simulink model "ddc_bpm_476_066"  (Simulink 7.8)
settings: Solver=ode45  StartTime=0.0  StopTime=2e-3  RelTol=1e-3
undefined symbols (not defined in the file): decim_factor_poly_35, dt_sim, frev_476, Fs_adc, n_ch, n_ovs, R_fofb, R_sec, R_sec_cfir, R_sec_pfir, R_tbt, xlipgetpartsetting
libraries: xbsIndex_r4 x1408, simulink x7
(part 8 of 11)

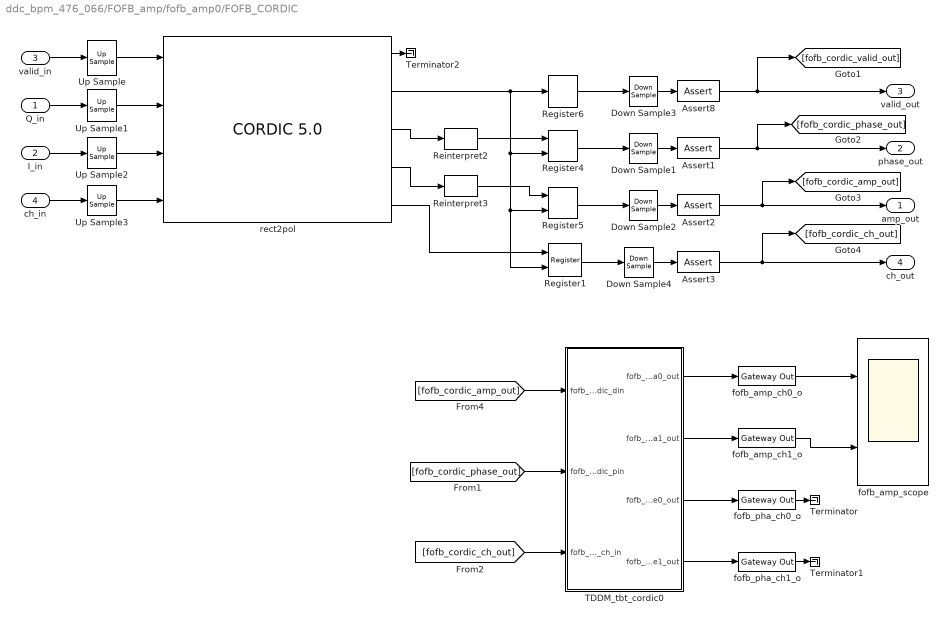
== system ddc_bpm_476_066/FOFB_amp/fofb_amp0/FOFB_CORDIC ==
  Q_in : Inport
  I_in : Inport  Port=2
  valid_in : Inport  Port=3
  ch_in : Inport  Port=4
  Assert{1..3,8} (4 alike) : xbsIndex_r4/Assert  assert_type=off  type_source=Explicitly  gui_display_data_type=Fixed-point  arith_type="Signed  (2's comp)"  n_bits=16  bin_pt=14  preci_type=Single  exp_width=8  frac_width=24  assert_rate=on  rate_source=Explicitly  period=(1/Fs_adc/n_ovs)*R_fofb  output_port=on  block_type=assert
  Down Sample{1..4} (4 alike) : xbsIndex_r4/Down Sample  sample_ratio=R_fofb  sample_phase="Last Value of Frame  (most efficient)"  en=off  latency=1  dbl_ovrd=off  block_type=dsamp
  Register1 : xbsIndex_r4/Register  init=0  rst=off  en=on  dbl_ovrd=off  block_type=register
  Register4 : xbsIndex_r4/Register  init=0  rst=off  en=on  dbl_ovrd=off  block_type=register
  Register5 : xbsIndex_r4/Register  init=0  rst=off  en=on  dbl_ovrd=off  block_type=register
  Register6 : xbsIndex_r4/Register  init=0  rst=off  en=off  dbl_ovrd=off  block_type=register
  Reinterpret2 : xbsIndex_r4/Reinterpret  force_arith_type=off  arith_type=Unsigned  force_bin_pt=off  bin_pt=18  block_type=reinterpret
  Reinterpret3 : xbsIndex_r4/Reinterpret  force_arith_type=off  arith_type=Unsigned  force_bin_pt=off  bin_pt=19  block_type=reinterpret
  TDDM_tbt_cordic0 : Subsystem
  Terminator : Terminator
  Terminator1 : Terminator
  Terminator2 : Terminator
  Up Sample : xbsIndex_r4/Up Sample  sample_ratio=R_fofb  copy_samples=off  en=off  latency=0  dbl_ovrd=off  block_type=usamp
  Up Sample1 : xbsIndex_r4/Up Sample  sample_ratio=R_fofb  copy_samples=on  en=off  latency=0  dbl_ovrd=off  block_type=usamp
  Up Sample2 : xbsIndex_r4/Up Sample  sample_ratio=R_fofb  copy_samples=on  en=off  latency=0  dbl_ovrd=off  block_type=usamp
  Up Sample3 : xbsIndex_r4/Up Sample  sample_ratio=R_fofb  copy_samples=on  en=off  latency=0  dbl_ovrd=off  block_type=usamp
  fofb_amp_ch0_o : xbsIndex_r4/Gateway Out  inherit_from_input=on  hdl_port=on  timing_constraint=Data Rate  locs_specified=off  LOCs={}  UseAsDAC=off  DACChannel='1'  block_type=gatewayout
      settings: infoedit="Gateway out block.  Converts Xilinx fixed-point or floating-point type inputs into ouputs of type Simulink integer, single, double, or fixed point.<br><br>Hardware notes:  In hardware these blocks become top level output ports or are discarded, depending on how they are configured."
  fofb_amp_ch1_o : xbsIndex_r4/Gateway Out  inherit_from_input=on  hdl_port=on  timing_constraint=Data Rate  locs_specified=off  LOCs={}  UseAsDAC=off  DACChannel='1'  block_type=gatewayout
      settings: infoedit="Gateway out block.  Converts Xilinx fixed-point or floating-point type inputs into ouputs of type Simulink integer, single, double, or fixed point.<br><br>Hardware notes:  In hardware these blocks become top level output ports or are discarded, depending on how they are configured."
  fofb_amp_scope : Scope  NumInputPorts=2
      settings: TimeRange=0.00011214  YMin=-0.1~-1.5  YMax=1~1.5  SaveName=ScopeData19  MaxDataPoints=1000000  SampleInput=on
  fofb_pha_ch0_o : xbsIndex_r4/Gateway Out  inherit_from_input=on  hdl_port=on  timing_constraint=Data Rate  locs_specified=off  LOCs={}  UseAsDAC=off  DACChannel='1'  block_type=gatewayout
      settings: infoedit="Gateway out block.  Converts Xilinx fixed-point or floating-point type inputs into ouputs of type Simulink integer, single, double, or fixed point.<br><br>Hardware notes:  In hardware these blocks become top level output ports or are discarded, depending on how they are configured."
  fofb_pha_ch1_o : xbsIndex_r4/Gateway Out  inherit_from_input=on  hdl_port=on  timing_constraint=Data Rate  locs_specified=off  LOCs={}  UseAsDAC=off  DACChannel='1'  block_type=gatewayout
      settings: infoedit="Gateway out block.  Converts Xilinx fixed-point or floating-point type inputs into ouputs of type Simulink integer, single, double, or fixed point.<br><br>Hardware notes:  In hardware these blocks become top level output ports or are discarded, depending on how they are configured."
  rect2pol : xbsIndex_r4/CORDIC 5.0   functional_selection=Translate  architectural_configuration=Word_Serial  pipelining_mode=Optimal  data_format=SignedFraction  phase_format=Radians  input_width=25  output_width=24  round_mode=Nearest_Even  iterations=0  precision=0  compensation_scaling=Embedded_Multiplier  coarse_rotation=on  aclken=off  aresetn=off  out_tready=off  cartesian_has_tuser=on  cartesian_has_tlast=off  cartesian_tuser_width=1  phase_has_tuser=off  phase_has_tlast=off  phase_tuser_width=1  out_tlast_behv=Null  flow_control=NonBlocking  optimize_goal=Resources  trim_axipin_name=on  ip_name=CORDIC  ip_version=5.0  dsptool_ready=true  ipcore_usecache=true  ipcore_useipmodelcache=true  wrapper_available=true  port_translation_map={ 'aclken' => 'en', 'aresetn' => 'rst' }  block_type=cordic_v5_0
      settings: infoedit=CORDIC 5.0
  amp_out : Outport
  phase_out : Outport  Port=2
  valid_out : Outport  Port=3
  ch_out : Outport  Port=4
  wires:
  Register4/1 -> Down Sample1/1
  Register5/1 -> Down Sample2/1
  Register6/1 -> Down Sample3/1
  [fofb_cordic_amp_out] -> TDDM_tbt_cordic0/1(fofb_cordic_din)
  [fofb_cordic_ch_out] -> TDDM_tbt_cordic0/3(fofb_cordic_ch_in)
  Register1/1 -> Down Sample4/1
  TDDM_tbt_cordic0/1(fofb_cordic_data0_out) -> fofb_amp_ch0_o/1
  TDDM_tbt_cordic0/2(fofb_cordic_data1_out) -> fofb_amp_ch1_o/1
  fofb_amp_ch0_o/1 -> fofb_amp_scope/1
  fofb_amp_ch1_o/1 -> fofb_amp_scope/2
  [fofb_cordic_phase_out] -> TDDM_tbt_cordic0/2(fofb_cordic_pin)
  TDDM_tbt_cordic0/3(fofb_cordic_phase0_out) -> fofb_pha_ch0_o/1
  TDDM_tbt_cordic0/4(fofb_cordic_phase1_out) -> fofb_pha_ch1_o/1
  fofb_pha_ch0_o/1 -> Terminator/1
  fofb_pha_ch1_o/1 -> Terminator1/1
  Reinterpret2/1 -> Register4/1
  Reinterpret3/1 -> Register5/1
  rect2pol/2 -> Register5/2, Register1/2, Register4/2, Register6/1
  rect2pol/3 -> Reinterpret2/1
  rect2pol/4 -> Reinterpret3/1
  rect2pol/5 -> Register1/1
  rect2pol/1 -> Terminator2/1
  valid_in/1 -> Up Sample/1
  Q_in/1 -> Up Sample1/1
  I_in/1 -> Up Sample2/1
  ch_in/1 -> Up Sample3/1
  Up Sample/1 -> rect2pol/1
  Up Sample1/1 -> rect2pol/2
  Up Sample2/1 -> rect2pol/3
  Up Sample3/1 -> rect2pol/4
  Down Sample3/1 -> Assert8/1
  Down Sample1/1 -> Assert1/1
  Down Sample2/1 -> Assert2/1
  Down Sample4/1 -> Assert3/1
  Assert8/1 -> valid_out/1, [fofb_cordic_valid_out]
  Assert1/1 -> phase_out/1, [fofb_cordic_phase_out]
  Assert2/1 -> amp_out/1, [fofb_cordic_amp_out]
  Assert3/1 -> ch_out/1, [fofb_cordic_ch_out]

== system ddc_bpm_476_066/FOFB_amp/fofb_amp0/FOFB_amp ==
  Q_in : Inport
  I_in : Inport  Port=2
  ch_in : Inport  Port=3
  Reg : Subsystem
  Reg1 : Subsystem
  TDDM_fofb_cic0 : Subsystem
  cic_fofb : Subsystem
  cic_fofb0_scope : Scope  NumInputPorts=4
      settings: TimeRange=0.00011214  YMin=-0.1~-1.5~-0.002~-1.5  YMax=1~1.5~0.00075~1.5  SaveName=ScopeData18  MaxDataPoints=1000000  SampleInput=on
  fofb_decim_ch0_i_o : xbsIndex_r4/Gateway Out  inherit_from_input=on  hdl_port=on  timing_constraint=Data Rate  locs_specified=off  LOCs={}  UseAsDAC=off  DACChannel='1'  block_type=gatewayout
      settings: infoedit="Gateway out block.  Converts Xilinx fixed-point or floating-point type inputs into ouputs of type Simulink integer, single, double, or fixed point.<br><br>Hardware notes:  In hardware these blocks become top level output ports or are discarded, depending on how they are configured."
  fofb_decim_ch0_q_o : xbsIndex_r4/Gateway Out  inherit_from_input=on  hdl_port=on  timing_constraint=Data Rate  locs_specified=off  LOCs={}  UseAsDAC=off  DACChannel='1'  block_type=gatewayout
      settings: infoedit="Gateway out block.  Converts Xilinx fixed-point or floating-point type inputs into ouputs of type Simulink integer, single, double, or fixed point.<br><br>Hardware notes:  In hardware these blocks become top level output ports or are discarded, depending on how they are configured."
  fofb_decim_ch1_i_o : xbsIndex_r4/Gateway Out  inherit_from_input=on  hdl_port=on  timing_constraint=Data Rate  locs_specified=off  LOCs={}  UseAsDAC=off  DACChannel='1'  block_type=gatewayout
      settings: infoedit="Gateway out block.  Converts Xilinx fixed-point or floating-point type inputs into ouputs of type Simulink integer, single, double, or fixed point.<br><br>Hardware notes:  In hardware these blocks become top level output ports or are discarded, depending on how they are configured."
  fofb_decim_ch1_q_o : xbsIndex_r4/Gateway Out  inherit_from_input=on  hdl_port=on  timing_constraint=Data Rate  locs_specified=off  LOCs={}  UseAsDAC=off  DACChannel='1'  block_type=gatewayout
      settings: infoedit="Gateway out block.  Converts Xilinx fixed-point or floating-point type inputs into ouputs of type Simulink integer, single, double, or fixed point.<br><br>Hardware notes:  In hardware these blocks become top level output ports or are discarded, depending on how they are configured."
  Q_out : Outport
  I_out : Outport  Port=2
  valid_out : Outport  Port=3
  ch_out : Outport  Port=4
  wires:
  Q_in/1 -> cic_fofb/2(Q_in)
  cic_fofb/1(Q_out) -> [fofb_cic_q_out], Q_out/1
  I_in/1 -> cic_fofb/3(I_in)
  cic_fofb/4(ch_out) -> ch_out/1, [fofb_cic_ch_out]
  ch_in/1 -> cic_fofb/1(ch_in)
  fofb_decim_ch1_q_o/1 -> cic_fofb0_scope/2
  fofb_decim_ch0_q_o/1 -> cic_fofb0_scope/1
  cic_fofb/3(valid_out) -> valid_out/1
  cic_fofb/2(I_out) -> [fofb_cic_i_out], I_out/1
  [fofb_cic_ch_out] -> TDDM_fofb_cic0/3(fofb_ch_in)
  Reg/1(dout) -> TDDM_fofb_cic0/1(fofb_q_in)
  Reg1/1(dout) -> TDDM_fofb_cic0/2(fofb_i_in)
  fofb_decim_ch0_i_o/1 -> cic_fofb0_scope/3
  fofb_decim_ch1_i_o/1 -> cic_fofb0_scope/4
  TDDM_fofb_cic0/4(cic_fofb_ch1_i_out) -> fofb_decim_ch1_i_o/1
  TDDM_fofb_cic0/1(cic_fofb_ch0_q_out) -> fofb_decim_ch0_q_o/1
  TDDM_fofb_cic0/2(cic_fofb_ch1_q_out) -> fofb_decim_ch1_q_o/1
  TDDM_fofb_cic0/3(cic_fofb_ch0_i_out) -> fofb_decim_ch0_i_o/1
  [fofb_cic_q_out] -> Reg/1(din)
  [fofb_cic_i_out] -> Reg1/1(din)

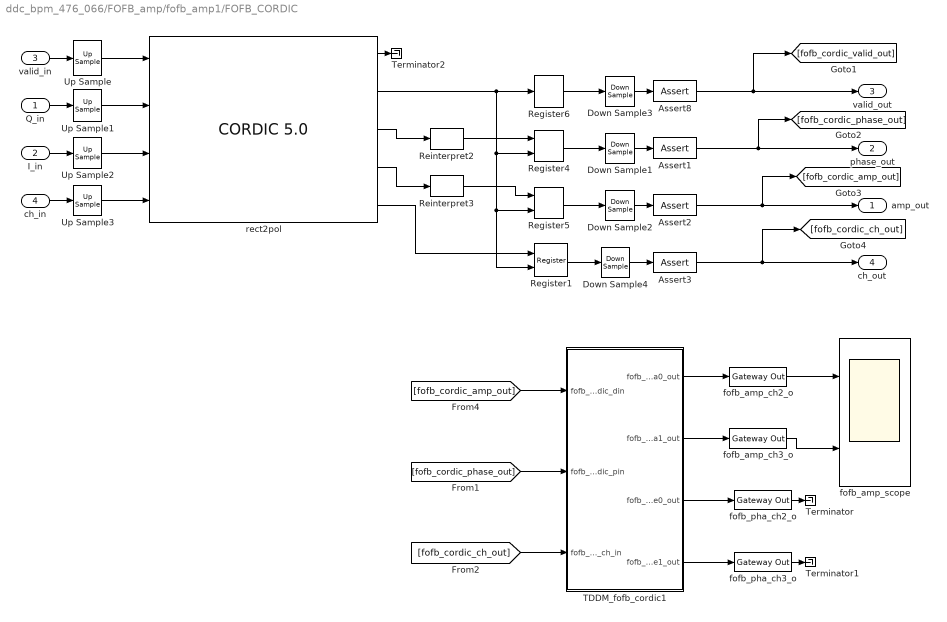
== system ddc_bpm_476_066/FOFB_amp/fofb_amp1/FOFB_CORDIC ==
  Q_in : Inport
  I_in : Inport  Port=2
  valid_in : Inport  Port=3
  ch_in : Inport  Port=4
  Assert{1..3,8} (4 alike) : xbsIndex_r4/Assert  assert_type=off  type_source=Explicitly  gui_display_data_type=Fixed-point  arith_type="Signed  (2's comp)"  n_bits=16  bin_pt=14  preci_type=Single  exp_width=8  frac_width=24  assert_rate=on  rate_source=Explicitly  period=(1/Fs_adc/n_ovs)*R_fofb  output_port=on  block_type=assert
  Down Sample{1..4} (4 alike) : xbsIndex_r4/Down Sample  sample_ratio=R_fofb  sample_phase="Last Value of Frame  (most efficient)"  en=off  latency=1  dbl_ovrd=off  block_type=dsamp
  Register1 : xbsIndex_r4/Register  init=0  rst=off  en=on  dbl_ovrd=off  block_type=register
  Register4 : xbsIndex_r4/Register  init=0  rst=off  en=on  dbl_ovrd=off  block_type=register
  Register5 : xbsIndex_r4/Register  init=0  rst=off  en=on  dbl_ovrd=off  block_type=register
  Register6 : xbsIndex_r4/Register  init=0  rst=off  en=off  dbl_ovrd=off  block_type=register
  Reinterpret2 : xbsIndex_r4/Reinterpret  force_arith_type=off  arith_type=Unsigned  force_bin_pt=off  bin_pt=18  block_type=reinterpret
  Reinterpret3 : xbsIndex_r4/Reinterpret  force_arith_type=off  arith_type=Unsigned  force_bin_pt=off  bin_pt=19  block_type=reinterpret
  TDDM_fofb_cordic1 : Subsystem
  Terminator : Terminator
  Terminator1 : Terminator
  Terminator2 : Terminator
  Up Sample : xbsIndex_r4/Up Sample  sample_ratio=R_fofb  copy_samples=off  en=off  latency=0  dbl_ovrd=off  block_type=usamp
  Up Sample1 : xbsIndex_r4/Up Sample  sample_ratio=R_fofb  copy_samples=on  en=off  latency=0  dbl_ovrd=off  block_type=usamp
  Up Sample2 : xbsIndex_r4/Up Sample  sample_ratio=R_fofb  copy_samples=on  en=off  latency=0  dbl_ovrd=off  block_type=usamp
  Up Sample3 : xbsIndex_r4/Up Sample  sample_ratio=R_fofb  copy_samples=on  en=off  latency=0  dbl_ovrd=off  block_type=usamp
  fofb_amp_ch2_o : xbsIndex_r4/Gateway Out  inherit_from_input=on  hdl_port=on  timing_constraint=Data Rate  locs_specified=off  LOCs={}  UseAsDAC=off  DACChannel='1'  block_type=gatewayout
      settings: infoedit="Gateway out block.  Converts Xilinx fixed-point or floating-point type inputs into ouputs of type Simulink integer, single, double, or fixed point.<br><br>Hardware notes:  In hardware these blocks become top level output ports or are discarded, depending on how they are configured."
  fofb_amp_ch3_o : xbsIndex_r4/Gateway Out  inherit_from_input=on  hdl_port=on  timing_constraint=Data Rate  locs_specified=off  LOCs={}  UseAsDAC=off  DACChannel='1'  block_type=gatewayout
      settings: infoedit="Gateway out block.  Converts Xilinx fixed-point or floating-point type inputs into ouputs of type Simulink integer, single, double, or fixed point.<br><br>Hardware notes:  In hardware these blocks become top level output ports or are discarded, depending on how they are configured."
  fofb_amp_scope : Scope  NumInputPorts=2
      settings: TimeRange=0.00011214  YMin=-0.1~-1.5  YMax=1~1.5  SaveName=ScopeData19  MaxDataPoints=1000000  SampleInput=on
  fofb_pha_ch2_o : xbsIndex_r4/Gateway Out  inherit_from_input=on  hdl_port=on  timing_constraint=Data Rate  locs_specified=off  LOCs={}  UseAsDAC=off  DACChannel='1'  block_type=gatewayout
      settings: infoedit="Gateway out block.  Converts Xilinx fixed-point or floating-point type inputs into ouputs of type Simulink integer, single, double, or fixed point.<br><br>Hardware notes:  In hardware these blocks become top level output ports or are discarded, depending on how they are configured."
  fofb_pha_ch3_o : xbsIndex_r4/Gateway Out  inherit_from_input=on  hdl_port=on  timing_constraint=Data Rate  locs_specified=off  LOCs={}  UseAsDAC=off  DACChannel='1'  block_type=gatewayout
      settings: infoedit="Gateway out block.  Converts Xilinx fixed-point or floating-point type inputs into ouputs of type Simulink integer, single, double, or fixed point.<br><br>Hardware notes:  In hardware these blocks become top level output ports or are discarded, depending on how they are configured."
  rect2pol : xbsIndex_r4/CORDIC 5.0   functional_selection=Translate  architectural_configuration=Word_Serial  pipelining_mode=Optimal  data_format=SignedFraction  phase_format=Radians  input_width=25  output_width=24  round_mode=Nearest_Even  iterations=0  precision=0  compensation_scaling=Embedded_Multiplier  coarse_rotation=on  aclken=off  aresetn=off  out_tready=off  cartesian_has_tuser=on  cartesian_has_tlast=off  cartesian_tuser_width=1  phase_has_tuser=off  phase_has_tlast=off  phase_tuser_width=1  out_tlast_behv=Null  flow_control=NonBlocking  optimize_goal=Resources  trim_axipin_name=on  ip_name=CORDIC  ip_version=5.0  dsptool_ready=true  ipcore_usecache=true  ipcore_useipmodelcache=true  wrapper_available=true  port_translation_map={ 'aclken' => 'en', 'aresetn' => 'rst' }  block_type=cordic_v5_0
      settings: infoedit=CORDIC 5.0
  amp_out : Outport
  phase_out : Outport  Port=2
  valid_out : Outport  Port=3
  ch_out : Outport  Port=4
  wires:
  [fofb_cordic_amp_out] -> TDDM_fofb_cordic1/1(fofb_cordic_din)
  [fofb_cordic_ch_out] -> TDDM_fofb_cordic1/3(fofb_cordic_ch_in)
  TDDM_fofb_cordic1/1(fofb_cordic_data0_out) -> fofb_amp_ch2_o/1
  TDDM_fofb_cordic1/2(fofb_cordic_data1_out) -> fofb_amp_ch3_o/1
  fofb_amp_ch2_o/1 -> fofb_amp_scope/1
  fofb_amp_ch3_o/1 -> fofb_amp_scope/2
  [fofb_cordic_phase_out] -> TDDM_fofb_cordic1/2(fofb_cordic_pin)
  TDDM_fofb_cordic1/3(fofb_cordic_phase0_out) -> fofb_pha_ch2_o/1
  TDDM_fofb_cordic1/4(fofb_cordic_phase1_out) -> fofb_pha_ch3_o/1
  fofb_pha_ch2_o/1 -> Terminator/1
  fofb_pha_ch3_o/1 -> Terminator1/1
  valid_in/1 -> Up Sample/1
  Q_in/1 -> Up Sample1/1
  I_in/1 -> Up Sample2/1
  ch_in/1 -> Up Sample3/1
  Register4/1 -> Down Sample1/1
  Register5/1 -> Down Sample2/1
  Register6/1 -> Down Sample3/1
  Register1/1 -> Down Sample4/1
  Reinterpret2/1 -> Register4/1
  Reinterpret3/1 -> Register5/1
  rect2pol/2 -> Register5/2, Register1/2, Register4/2, Register6/1
  rect2pol/3 -> Reinterpret2/1
  rect2pol/4 -> Reinterpret3/1
  rect2pol/5 -> Register1/1
  rect2pol/1 -> Terminator2/1
  Up Sample/1 -> rect2pol/1
  Up Sample1/1 -> rect2pol/2
  Up Sample2/1 -> rect2pol/3
  Up Sample3/1 -> rect2pol/4
  Down Sample3/1 -> Assert8/1
  Down Sample1/1 -> Assert1/1
  Down Sample2/1 -> Assert2/1
  Down Sample4/1 -> Assert3/1
  Assert8/1 -> valid_out/1, [fofb_cordic_valid_out]
  Assert1/1 -> phase_out/1, [fofb_cordic_phase_out]
  Assert2/1 -> amp_out/1, [fofb_cordic_amp_out]
  Assert3/1 -> ch_out/1, [fofb_cordic_ch_out]

== system ddc_bpm_476_066/FOFB_amp/fofb_amp1/FOFB_amp ==
  Q_in : Inport
  I_in : Inport  Port=2
  ch_in : Inport  Port=3
  Reg : Subsystem
  Reg1 : Subsystem
  TDDM_fofb_cic1 : Subsystem
  cic_fofb : Subsystem
  cic_fofb0_scope : Scope  NumInputPorts=4
      settings: TimeRange=0.00011214  YMin=-0.1~-1.5~-0.002~-1.5  YMax=1~1.5~0.00075~1.5  SaveName=ScopeData18  MaxDataPoints=1000000  SampleInput=on
  fofb_decim_ch2_i_o : xbsIndex_r4/Gateway Out  inherit_from_input=on  hdl_port=on  timing_constraint=Data Rate  locs_specified=off  LOCs={}  UseAsDAC=off  DACChannel='1'  block_type=gatewayout
      settings: infoedit="Gateway out block.  Converts Xilinx fixed-point or floating-point type inputs into ouputs of type Simulink integer, single, double, or fixed point.<br><br>Hardware notes:  In hardware these blocks become top level output ports or are discarded, depending on how they are configured."
  fofb_decim_ch2_q_o : xbsIndex_r4/Gateway Out  inherit_from_input=on  hdl_port=on  timing_constraint=Data Rate  locs_specified=off  LOCs={}  UseAsDAC=off  DACChannel='1'  block_type=gatewayout
      settings: infoedit="Gateway out block.  Converts Xilinx fixed-point or floating-point type inputs into ouputs of type Simulink integer, single, double, or fixed point.<br><br>Hardware notes:  In hardware these blocks become top level output ports or are discarded, depending on how they are configured."
  fofb_decim_ch3_i_o : xbsIndex_r4/Gateway Out  inherit_from_input=on  hdl_port=on  timing_constraint=Data Rate  locs_specified=off  LOCs={}  UseAsDAC=off  DACChannel='1'  block_type=gatewayout
      settings: infoedit="Gateway out block.  Converts Xilinx fixed-point or floating-point type inputs into ouputs of type Simulink integer, single, double, or fixed point.<br><br>Hardware notes:  In hardware these blocks become top level output ports or are discarded, depending on how they are configured."
  fofb_decim_ch3_q_o : xbsIndex_r4/Gateway Out  inherit_from_input=on  hdl_port=on  timing_constraint=Data Rate  locs_specified=off  LOCs={}  UseAsDAC=off  DACChannel='1'  block_type=gatewayout
      settings: infoedit="Gateway out block.  Converts Xilinx fixed-point or floating-point type inputs into ouputs of type Simulink integer, single, double, or fixed point.<br><br>Hardware notes:  In hardware these blocks become top level output ports or are discarded, depending on how they are configured."
  Q_out : Outport
  I_out : Outport  Port=2
  valid_out : Outport  Port=3
  ch_out : Outport  Port=4
  wires:
  Q_in/1 -> cic_fofb/2(Q_in)
  cic_fofb/1(Q_out) -> [fofb_cic_q_out], Q_out/1
  I_in/1 -> cic_fofb/3(I_in)
  cic_fofb/4(ch_out) -> ch_out/1, [fofb_cic_ch_out]
  ch_in/1 -> cic_fofb/1(ch_in)
  fofb_decim_ch3_q_o/1 -> cic_fofb0_scope/2
  fofb_decim_ch2_q_o/1 -> cic_fofb0_scope/1
  cic_fofb/3(valid_out) -> valid_out/1
  cic_fofb/2(I_out) -> [fofb_cic_i_out], I_out/1
  [fofb_cic_ch_out] -> TDDM_fofb_cic1/3(fofb_ch_in)
  Reg/1(dout) -> TDDM_fofb_cic1/1(fofb_q_in)
  Reg1/1(dout) -> TDDM_fofb_cic1/2(fofb_i_in)
  fofb_decim_ch2_i_o/1 -> cic_fofb0_scope/3
  fofb_decim_ch3_i_o/1 -> cic_fofb0_scope/4
  TDDM_fofb_cic1/4(cic_fofb_ch1_i_out) -> fofb_decim_ch3_i_o/1
  TDDM_fofb_cic1/1(cic_fofb_ch0_q_out) -> fofb_decim_ch2_q_o/1
  TDDM_fofb_cic1/2(cic_fofb_ch1_q_out) -> fofb_decim_ch3_q_o/1
  TDDM_fofb_cic1/3(cic_fofb_ch0_i_out) -> fofb_decim_ch2_i_o/1
  [fofb_cic_q_out] -> Reg/1(din)
  [fofb_cic_i_out] -> Reg1/1(din)

== system ddc_bpm_476_066/Mixer/CMixer_0/DataReg_En ==
  Din : Inport
  en : Inport  Port=2
  Register : xbsIndex_r4/Register  init=0  rst=off  en=on  dbl_ovrd=off  block_type=register
      settings: block_version=VER_STRING_GOES_HERE
  Register1 : xbsIndex_r4/Register  init=0  rst=off  en=off  dbl_ovrd=off  block_type=register
      settings: block_version=VER_STRING_GOES_HERE
  Dout : Outport
  Valid : Outport  Port=2
  wires:
  Din/1 -> Register/1
  Register/1 -> Dout/1
  Register1/1 -> Valid/1
  en/1 -> Register1/1, Register/2

== system ddc_bpm_476_066/Mixer/CMixer_0/DataReg_En1 ==
  Din : Inport
  en : Inport  Port=2
  Register : xbsIndex_r4/Register  init=0  rst=off  en=on  dbl_ovrd=off  block_type=register
      settings: block_version=VER_STRING_GOES_HERE
  Register1 : xbsIndex_r4/Register  init=0  rst=off  en=off  dbl_ovrd=off  block_type=register
      settings: block_version=VER_STRING_GOES_HERE
  Dout : Outport
  Valid : Outport  Port=2
  wires:
  Din/1 -> Register/1
  Register/1 -> Dout/1
  Register1/1 -> Valid/1
  en/1 -> Register1/1, Register/2

== system ddc_bpm_476_066/Mixer/CMixer_1/DataReg_En ==
  Din : Inport
  en : Inport  Port=2
  Register : xbsIndex_r4/Register  init=0  rst=off  en=on  dbl_ovrd=off  block_type=register
      settings: block_version=VER_STRING_GOES_HERE
  Register1 : xbsIndex_r4/Register  init=0  rst=off  en=off  dbl_ovrd=off  block_type=register
      settings: block_version=VER_STRING_GOES_HERE
  Dout : Outport
  Valid : Outport  Port=2
  wires:
  Din/1 -> Register/1
  Register/1 -> Dout/1
  Register1/1 -> Valid/1
  en/1 -> Register1/1, Register/2

== system ddc_bpm_476_066/Mixer/CMixer_1/DataReg_En1 ==
  Din : Inport
  en : Inport  Port=2
  Register : xbsIndex_r4/Register  init=0  rst=off  en=on  dbl_ovrd=off  block_type=register
      settings: block_version=VER_STRING_GOES_HERE
  Register1 : xbsIndex_r4/Register  init=0  rst=off  en=off  dbl_ovrd=off  block_type=register
      settings: block_version=VER_STRING_GOES_HERE
  Dout : Outport
  Valid : Outport  Port=2
  wires:
  Din/1 -> Register/1
  Register/1 -> Dout/1
  Register1/1 -> Valid/1
  en/1 -> Register1/1, Register/2

== system ddc_bpm_476_066/Mixer/TDDM_Mixer/TDDM_Mixer0_i ==
  din : Inport
  ch_in : Inport  Port=2
  Constant : xbsIndex_r4/Constant  const=1  gui_display_data_type=Fixed-point  arith_type=Unsigned  n_bits=1  bin_pt=0  preci_type=Single  exp_width=8  frac_width=24  explicit_period=off  period=1  equ=P=C  opselect=C  inp2=PCIN>>17  opr=+  inp1=P  carry=CIN  dbl_ovrd=off  block_type=constant
  Constant1 : xbsIndex_r4/Constant  const=0  gui_display_data_type=Fixed-point  arith_type=Unsigned  n_bits=2  bin_pt=0  preci_type=Single  exp_width=8  frac_width=24  explicit_period=off  period=1  equ=P=C  opselect=C  inp2=PCIN>>17  opr=+  inp1=P  carry=CIN  dbl_ovrd=off  block_type=constant
  Delay : xbsIndex_r4/Delay  rst=off  infoeditControl=Selection of Reset will increase slice count due to use of real FFs and instead of SRLs  en=off  latency=3  dbl_ovrd=off  reg_retiming=off  block_type=delay
  Down Sample1 : xbsIndex_r4/Down Sample  sample_ratio=n_ch/n_ovs  sample_phase="Last Value of Frame  (most efficient)"  en=off  latency=1  dbl_ovrd=off  block_type=dsamp
  Down Sample2 : xbsIndex_r4/Down Sample  sample_ratio=n_ch/n_ovs  sample_phase="Last Value of Frame  (most efficient)"  en=off  latency=1  dbl_ovrd=off  block_type=dsamp
  Register : xbsIndex_r4/Register  init=0  rst=off  en=on  dbl_ovrd=off  block_type=register
  Register1 : xbsIndex_r4/Register  init=0  rst=off  en=on  dbl_ovrd=off  block_type=register
  Relational : xbsIndex_r4/Relational  mode=a=b  en=off  latency=1  dbl_ovrd=off  block_type=relational
  Relational1 : xbsIndex_r4/Relational  mode=a=b  en=off  latency=1  dbl_ovrd=off  block_type=relational
  dout_ch0 : Outport
  dout_ch1 : Outport  Port=2
  ch_out : Outport  Port=3
  wires:
  Constant/1 -> Relational/2
  Constant1/1 -> Relational1/2
  Relational/1 -> Register/2
  Relational1/1 -> Register1/2
  din/1 -> Register/1, Register1/1
  Register/1 -> Down Sample2/1
  ch_in/1 -> Relational/1, Relational1/1, Delay/1
  Register1/1 -> Down Sample1/1
  Down Sample2/1 -> dout_ch0/1
  Delay/1 -> ch_out/1
  Down Sample1/1 -> dout_ch1/1

== system ddc_bpm_476_066/Mixer/TDDM_Mixer/TDDM_Mixer0_q ==
  din : Inport
  ch_in : Inport  Port=2
  Constant : xbsIndex_r4/Constant  const=1  gui_display_data_type=Fixed-point  arith_type=Unsigned  n_bits=1  bin_pt=0  preci_type=Single  exp_width=8  frac_width=24  explicit_period=off  period=1  equ=P=C  opselect=C  inp2=PCIN>>17  opr=+  inp1=P  carry=CIN  dbl_ovrd=off  block_type=constant
  Constant1 : xbsIndex_r4/Constant  const=0  gui_display_data_type=Fixed-point  arith_type=Unsigned  n_bits=2  bin_pt=0  preci_type=Single  exp_width=8  frac_width=24  explicit_period=off  period=1  equ=P=C  opselect=C  inp2=PCIN>>17  opr=+  inp1=P  carry=CIN  dbl_ovrd=off  block_type=constant
  Delay : xbsIndex_r4/Delay  rst=off  infoeditControl=Selection of Reset will increase slice count due to use of real FFs and instead of SRLs  en=off  latency=3  dbl_ovrd=off  reg_retiming=off  block_type=delay
  Down Sample1 : xbsIndex_r4/Down Sample  sample_ratio=n_ch/n_ovs  sample_phase="Last Value of Frame  (most efficient)"  en=off  latency=1  dbl_ovrd=off  block_type=dsamp
  Down Sample2 : xbsIndex_r4/Down Sample  sample_ratio=n_ch/n_ovs  sample_phase="Last Value of Frame  (most efficient)"  en=off  latency=1  dbl_ovrd=off  block_type=dsamp
  Register : xbsIndex_r4/Register  init=0  rst=off  en=on  dbl_ovrd=off  block_type=register
  Register1 : xbsIndex_r4/Register  init=0  rst=off  en=on  dbl_ovrd=off  block_type=register
  Relational : xbsIndex_r4/Relational  mode=a=b  en=off  latency=1  dbl_ovrd=off  block_type=relational
  Relational1 : xbsIndex_r4/Relational  mode=a=b  en=off  latency=1  dbl_ovrd=off  block_type=relational
  dout_ch0 : Outport
  dout_ch1 : Outport  Port=2
  ch_out : Outport  Port=3
  wires:
  Constant/1 -> Relational/2
  Constant1/1 -> Relational1/2
  Relational/1 -> Register/2
  Relational1/1 -> Register1/2
  din/1 -> Register/1, Register1/1
  Register/1 -> Down Sample2/1
  ch_in/1 -> Relational/1, Relational1/1, Delay/1
  Register1/1 -> Down Sample1/1
  Down Sample2/1 -> dout_ch0/1
  Delay/1 -> ch_out/1
  Down Sample1/1 -> dout_ch1/1

== system ddc_bpm_476_066/Mixer/TDDM_Mixer/TDDM_Mixer1_i ==
  din : Inport
  ch_in : Inport  Port=2
  Constant : xbsIndex_r4/Constant  const=1  gui_display_data_type=Fixed-point  arith_type=Unsigned  n_bits=1  bin_pt=0  preci_type=Single  exp_width=8  frac_width=24  explicit_period=off  period=1  equ=P=C  opselect=C  inp2=PCIN>>17  opr=+  inp1=P  carry=CIN  dbl_ovrd=off  block_type=constant
  Constant1 : xbsIndex_r4/Constant  const=0  gui_display_data_type=Fixed-point  arith_type=Unsigned  n_bits=2  bin_pt=0  preci_type=Single  exp_width=8  frac_width=24  explicit_period=off  period=1  equ=P=C  opselect=C  inp2=PCIN>>17  opr=+  inp1=P  carry=CIN  dbl_ovrd=off  block_type=constant
  Delay : xbsIndex_r4/Delay  rst=off  infoeditControl=Selection of Reset will increase slice count due to use of real FFs and instead of SRLs  en=off  latency=3  dbl_ovrd=off  reg_retiming=off  block_type=delay
  Down Sample1 : xbsIndex_r4/Down Sample  sample_ratio=n_ch/n_ovs  sample_phase="Last Value of Frame  (most efficient)"  en=off  latency=1  dbl_ovrd=off  block_type=dsamp
  Down Sample2 : xbsIndex_r4/Down Sample  sample_ratio=n_ch/n_ovs  sample_phase="Last Value of Frame  (most efficient)"  en=off  latency=1  dbl_ovrd=off  block_type=dsamp
  Register : xbsIndex_r4/Register  init=0  rst=off  en=on  dbl_ovrd=off  block_type=register
  Register1 : xbsIndex_r4/Register  init=0  rst=off  en=on  dbl_ovrd=off  block_type=register
  Relational : xbsIndex_r4/Relational  mode=a=b  en=off  latency=1  dbl_ovrd=off  block_type=relational
  Relational1 : xbsIndex_r4/Relational  mode=a=b  en=off  latency=1  dbl_ovrd=off  block_type=relational
  dout_ch0 : Outport
  dout_ch1 : Outport  Port=2
  ch_out : Outport  Port=3
  wires:
  Constant/1 -> Relational/2
  Constant1/1 -> Relational1/2
  Relational/1 -> Register/2
  Relational1/1 -> Register1/2
  din/1 -> Register/1, Register1/1
  Register/1 -> Down Sample2/1
  ch_in/1 -> Relational/1, Relational1/1, Delay/1
  Register1/1 -> Down Sample1/1
  Down Sample2/1 -> dout_ch0/1
  Delay/1 -> ch_out/1
  Down Sample1/1 -> dout_ch1/1

== system ddc_bpm_476_066/Mixer/TDDM_Mixer/TDDM_Mixer1_q ==
  din : Inport
  ch_in : Inport  Port=2
  Constant : xbsIndex_r4/Constant  const=1  gui_display_data_type=Fixed-point  arith_type=Unsigned  n_bits=1  bin_pt=0  preci_type=Single  exp_width=8  frac_width=24  explicit_period=off  period=1  equ=P=C  opselect=C  inp2=PCIN>>17  opr=+  inp1=P  carry=CIN  dbl_ovrd=off  block_type=constant
  Constant1 : xbsIndex_r4/Constant  const=0  gui_display_data_type=Fixed-point  arith_type=Unsigned  n_bits=2  bin_pt=0  preci_type=Single  exp_width=8  frac_width=24  explicit_period=off  period=1  equ=P=C  opselect=C  inp2=PCIN>>17  opr=+  inp1=P  carry=CIN  dbl_ovrd=off  block_type=constant
  Delay : xbsIndex_r4/Delay  rst=off  infoeditControl=Selection of Reset will increase slice count due to use of real FFs and instead of SRLs  en=off  latency=3  dbl_ovrd=off  reg_retiming=off  block_type=delay
  Down Sample1 : xbsIndex_r4/Down Sample  sample_ratio=n_ch/n_ovs  sample_phase="Last Value of Frame  (most efficient)"  en=off  latency=1  dbl_ovrd=off  block_type=dsamp
  Down Sample2 : xbsIndex_r4/Down Sample  sample_ratio=n_ch/n_ovs  sample_phase="Last Value of Frame  (most efficient)"  en=off  latency=1  dbl_ovrd=off  block_type=dsamp
  Register : xbsIndex_r4/Register  init=0  rst=off  en=on  dbl_ovrd=off  block_type=register
  Register1 : xbsIndex_r4/Register  init=0  rst=off  en=on  dbl_ovrd=off  block_type=register
  Relational : xbsIndex_r4/Relational  mode=a=b  en=off  latency=1  dbl_ovrd=off  block_type=relational
  Relational1 : xbsIndex_r4/Relational  mode=a=b  en=off  latency=1  dbl_ovrd=off  block_type=relational
  dout_ch0 : Outport
  dout_ch1 : Outport  Port=2
  ch_out : Outport  Port=3
  wires:
  Constant/1 -> Relational/2
  Constant1/1 -> Relational1/2
  Relational/1 -> Register/2
  Relational1/1 -> Register1/2
  din/1 -> Register/1, Register1/1
  Register/1 -> Down Sample2/1
  ch_in/1 -> Relational/1, Relational1/1, Delay/1
  Register1/1 -> Down Sample1/1
  Down Sample2/1 -> dout_ch0/1
  Delay/1 -> ch_out/1
  Down Sample1/1 -> dout_ch1/1

== system ddc_bpm_476_066/Monit_amp/Monit_amp_c/Cast2 ==
  data_in : Inport
  en : Inport  Port=2
  Register : xbsIndex_r4/Register  init=0  rst=off  en=on  dbl_ovrd=off  block_type=register
      settings: xl_area=[0, 0, 0, 0, 0, 0, 0]  block_version=VER_STRING_GOES_HERE
  Register1 : xbsIndex_r4/Register  init=0  rst=off  en=off  dbl_ovrd=off  block_type=register
      settings: xl_area=[0, 0, 0, 0, 0, 0, 0]  block_version=VER_STRING_GOES_HERE
  format1 : Subsystem
  out : Outport
  valid : Outport  Port=2
  wires:
  format1/1(dout) -> Register/1
  Register/1 -> out/1
  en/1 -> Register/2, Register1/1
  data_in/1 -> format1/1(din)
  Register1/1 -> valid/1

== system ddc_bpm_476_066/Monit_amp/Monit_amp_c/Cast4 ==
  data_in : Inport
  en : Inport  Port=2
  Register : xbsIndex_r4/Register  init=0  rst=off  en=on  dbl_ovrd=off  block_type=register
      settings: xl_area=[0, 0, 0, 0, 0, 0, 0]  block_version=VER_STRING_GOES_HERE
  format1 : Subsystem
  out : Outport
  wires:
  format1/1(dout) -> Register/1
  Register/1 -> out/1
  en/1 -> Register/2
  data_in/1 -> format1/1(din)

== system ddc_bpm_476_066/Monit_amp/Monit_amp_c/Reg1 ==
  din : Inport
  en : Inport  Port=2
  Convert : xbsIndex_r4/Convert  gui_display_data_type=Fixed-point  arith_type="Signed  (2's comp)"  n_bits=24  bin_pt=22  float_type=Single  exp_bits=8  fraction_bits=24  quantization="Round  (unbiased: +/- Inf)"  overflow=Flag as error  en=off  latency=0  dbl_ovrd=off  pipeline=off  block_type=convert
  Register : xbsIndex_r4/Register  init=0  rst=off  en=on  dbl_ovrd=off  block_type=register
      settings: xl_area=[0, 0, 0, 0, 0, 0, 0]  block_version=VER_STRING_GOES_HERE
  Register1 : xbsIndex_r4/Register  init=0  rst=off  en=off  dbl_ovrd=off  block_type=register
      settings: xl_area=[0, 0, 0, 0, 0, 0, 0]  block_version=VER_STRING_GOES_HERE
  Reinterpret2 : xbsIndex_r4/Reinterpret  force_arith_type=on  arith_type="Signed  (2's comp)"  force_bin_pt=on  bin_pt=59  block_type=cast
      settings: block_version=VER_STRING_GOES_HERE
  dout : Outport
  valid_out : Outport  Port=2
  wires:
  Register/1 -> dout/1
  en/1 -> Register/2, Register1/1
  din/1 -> Reinterpret2/1
  Reinterpret2/1 -> Convert/1
  Register1/1 -> valid_out/1
  Convert/1 -> Register/1

== system ddc_bpm_476_066/Monit_amp/Monit_amp_c/ST2 ==
  In : Inport
  Display : Display
  Sample Time : xbsIndex_r4/Sample Time  block_type=sampletime
      settings: infoedit="The Sample Time block reports the normalized sample period of its input.  A signal's normalized sample period is not equivalent to its Simulink absolute sample period.<br><br>Hardware notes: This block is implemented as a constant in hardware."
  X_monit1 : xbsIndex_r4/Gateway Out  inherit_from_input=on  hdl_port=off  timing_constraint=Data Rate  locs_specified=off  LOCs={}  UseAsDAC=off  DACChannel='1'  block_type=gatewayout
      settings: infoedit="Gateway out block.  Converts Xilinx fixed-point or floating-point type inputs into ouputs of type Simulink integer, single, double, or fixed point.<br><br>Hardware notes:  In hardware these blocks become top level output ports or are discarded, depending on how they are configured."
  wires:
  X_monit1/1 -> Display/1
  Sample Time/1 -> X_monit1/1
  In/1 -> Sample Time/1

== system ddc_bpm_476_066/Monit_amp/Monit_amp_c/ST3 ==
  In : Inport
  Display : Display
  Sample Time : xbsIndex_r4/Sample Time  block_type=sampletime
      settings: infoedit="The Sample Time block reports the normalized sample period of its input.  A signal's normalized sample period is not equivalent to its Simulink absolute sample period.<br><br>Hardware notes: This block is implemented as a constant in hardware."
  X_monit1 : xbsIndex_r4/Gateway Out  inherit_from_input=on  hdl_port=off  timing_constraint=Data Rate  locs_specified=off  LOCs={}  UseAsDAC=off  DACChannel='1'  block_type=gatewayout
      settings: infoedit="Gateway out block.  Converts Xilinx fixed-point or floating-point type inputs into ouputs of type Simulink integer, single, double, or fixed point.<br><br>Hardware notes:  In hardware these blocks become top level output ports or are discarded, depending on how they are configured."
  wires:
  X_monit1/1 -> Display/1
  Sample Time/1 -> X_monit1/1
  In/1 -> Sample Time/1

== system ddc_bpm_476_066/Monit_amp/Monit_amp_c/ST4 ==
  In : Inport
  Display : Display
  Sample Time : xbsIndex_r4/Sample Time  block_type=sampletime
      settings: infoedit="The Sample Time block reports the normalized sample period of its input.  A signal's normalized sample period is not equivalent to its Simulink absolute sample period.<br><br>Hardware notes: This block is implemented as a constant in hardware."
  X_monit1 : xbsIndex_r4/Gateway Out  inherit_from_input=on  hdl_port=off  timing_constraint=Data Rate  locs_specified=off  LOCs={}  UseAsDAC=off  DACChannel='1'  block_type=gatewayout
      settings: infoedit="Gateway out block.  Converts Xilinx fixed-point or floating-point type inputs into ouputs of type Simulink integer, single, double, or fixed point.<br><br>Hardware notes:  In hardware these blocks become top level output ports or are discarded, depending on how they are configured."
  wires:
  X_monit1/1 -> Display/1
  Sample Time/1 -> X_monit1/1
  In/1 -> Sample Time/1

== system ddc_bpm_476_066/Monit_amp/Monit_amp_c/ST5 ==
  In : Inport
  Display : Display
  Sample Time : xbsIndex_r4/Sample Time  block_type=sampletime
      settings: infoedit="The Sample Time block reports the normalized sample period of its input.  A signal's normalized sample period is not equivalent to its Simulink absolute sample period.<br><br>Hardware notes: This block is implemented as a constant in hardware."
  X_monit1 : xbsIndex_r4/Gateway Out  inherit_from_input=on  hdl_port=off  timing_constraint=Data Rate  locs_specified=off  LOCs={}  UseAsDAC=off  DACChannel='1'  block_type=gatewayout
      settings: infoedit="Gateway out block.  Converts Xilinx fixed-point or floating-point type inputs into ouputs of type Simulink integer, single, double, or fixed point.<br><br>Hardware notes:  In hardware these blocks become top level output ports or are discarded, depending on how they are configured."
  wires:
  X_monit1/1 -> Display/1
  Sample Time/1 -> X_monit1/1
  In/1 -> Sample Time/1

== system ddc_bpm_476_066/Monit_amp/Monit_amp_c/TDDM_monit_amp_c ==
  monit_din : Inport
  monit_ch_in : Inport  Port=2
  TDDM_monit_amp_c_int : Subsystem
  Terminator : Terminator
  monit_ch0_out : Outport
  monit_ch1_out : Outport  Port=2
  monit_ch2_out : Outport  Port=3
  monit_ch3_out : Outport  Port=4
  wires:
  monit_din/1 -> TDDM_monit_amp_c_int/1(din)
  monit_ch_in/1 -> TDDM_monit_amp_c_int/2(ch_in)
  TDDM_monit_amp_c_int/1(dout_ch0) -> monit_ch0_out/1
  TDDM_monit_amp_c_int/2(dout_ch1) -> monit_ch1_out/1
  TDDM_monit_amp_c_int/3(dout_ch2) -> monit_ch2_out/1
  TDDM_monit_amp_c_int/4(dout_ch3) -> monit_ch3_out/1
  TDDM_monit_amp_c_int/5(ch_out) -> Terminator/1

== system ddc_bpm_476_066/Monit_amp/TDDM_monit_amp_out/TDDM_monit_amp_out_int ==
  din : Inport
  ch_in : Inport  Port=2
  Constant : xbsIndex_r4/Constant  const=3  gui_display_data_type=Fixed-point  arith_type=Unsigned  n_bits=2  bin_pt=0  preci_type=Single  exp_width=8  frac_width=24  explicit_period=off  period=1  equ=P=C  opselect=C  inp2=PCIN>>17  opr=+  inp1=P  carry=CIN  dbl_ovrd=off  block_type=constant
  Constant1 : xbsIndex_r4/Constant  const=0  gui_display_data_type=Fixed-point  arith_type=Unsigned  n_bits=2  bin_pt=0  preci_type=Single  exp_width=8  frac_width=24  explicit_period=off  period=1  equ=P=C  opselect=C  inp2=PCIN>>17  opr=+  inp1=P  carry=CIN  dbl_ovrd=off  block_type=constant
  Constant3 : xbsIndex_r4/Constant  const=1  gui_display_data_type=Fixed-point  arith_type=Unsigned  n_bits=2  bin_pt=0  preci_type=Single  exp_width=8  frac_width=24  explicit_period=off  period=1  equ=P=C  opselect=C  inp2=PCIN>>17  opr=+  inp1=P  carry=CIN  dbl_ovrd=off  block_type=constant
  Constant4 : xbsIndex_r4/Constant  const=2  gui_display_data_type=Fixed-point  arith_type=Unsigned  n_bits=2  bin_pt=0  preci_type=Single  exp_width=8  frac_width=24  explicit_period=off  period=1  equ=P=C  opselect=C  inp2=PCIN>>17  opr=+  inp1=P  carry=CIN  dbl_ovrd=off  block_type=constant
  Delay : xbsIndex_r4/Delay  rst=off  infoeditControl=Selection of Reset will increase slice count due to use of real FFs and instead of SRLs  en=off  latency=3  dbl_ovrd=off  reg_retiming=off  block_type=delay
  Down Sample{1..4} (4 alike) : xbsIndex_r4/Down Sample  sample_ratio=n_ch  sample_phase="Last Value of Frame  (most efficient)"  en=off  latency=1  dbl_ovrd=off  block_type=dsamp
  Register{,1..3} (4 alike) : xbsIndex_r4/Register  init=0  rst=off  en=on  dbl_ovrd=off  block_type=register
  Relational{,1..3} (4 alike) : xbsIndex_r4/Relational  mode=a=b  en=off  latency=1  dbl_ovrd=off  block_type=relational
  dout_ch0 : Outport
  dout_ch1 : Outport  Port=2
  dout_ch2 : Outport  Port=3
  dout_ch3 : Outport  Port=4
  ch_out : Outport  Port=5
  wires:
  Constant/1 -> Relational/2
  Constant1/1 -> Relational1/2
  Constant3/1 -> Relational2/2
  Constant4/1 -> Relational3/2
  Relational/1 -> Register/2
  Relational1/1 -> Register1/2
  Relational2/1 -> Register2/2
  Relational3/1 -> Register3/2
  din/1 -> Register1/1, Register2/1, Register3/1, Register/1
  Register/1 -> Down Sample2/1
  ch_in/1 -> Relational/1, Relational1/1, Relational2/1, Relational3/1, Delay/1
  Register1/1 -> Down Sample1/1
  Register2/1 -> Down Sample3/1
  Register3/1 -> Down Sample4/1
  Down Sample2/1 -> dout_ch0/1
  Delay/1 -> ch_out/1
  Down Sample3/1 -> dout_ch2/1
  Down Sample1/1 -> dout_ch1/1
  Down Sample4/1 -> dout_ch3/1

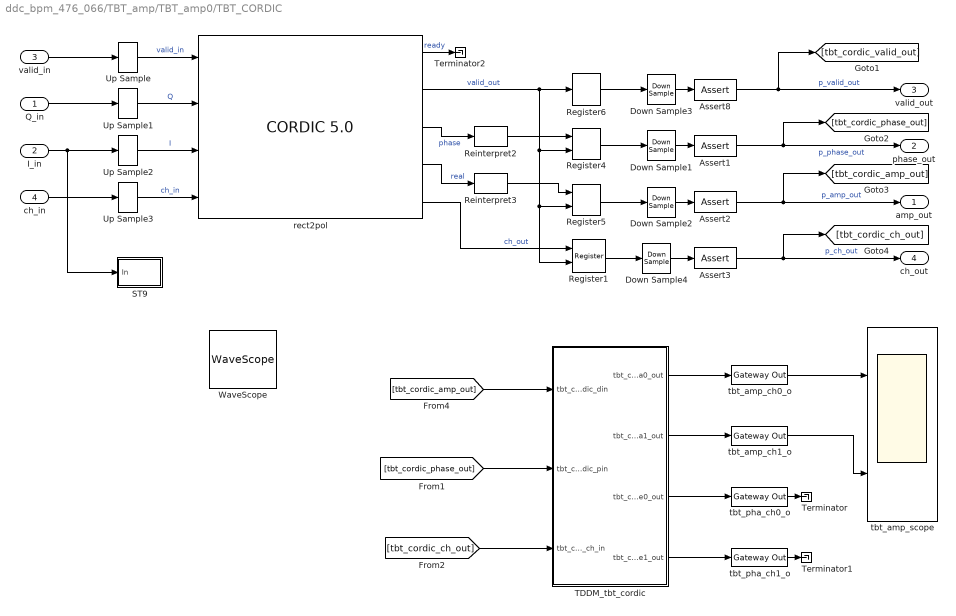
== system ddc_bpm_476_066/TBT_amp/TBT_amp0/TBT_CORDIC ==
  Q_in : Inport
  I_in : Inport  Port=2
  valid_in : Inport  Port=3
  ch_in : Inport  Port=4
  Assert{1..3,8} (4 alike) : xbsIndex_r4/Assert  assert_type=off  type_source=Explicitly  gui_display_data_type=Fixed-point  arith_type="Signed  (2's comp)"  n_bits=16  bin_pt=14  preci_type=Single  exp_width=8  frac_width=24  assert_rate=on  rate_source=Explicitly  period=(1/Fs_adc/n_ovs)*decim_factor_poly_35  output_port=on  block_type=assert
  Down Sample{1..4} (4 alike) : xbsIndex_r4/Down Sample  sample_ratio=decim_factor_poly_35  sample_phase="Last Value of Frame  (most efficient)"  en=off  latency=1  dbl_ovrd=off  block_type=dsamp
  Register1 : xbsIndex_r4/Register  init=0  rst=off  en=on  dbl_ovrd=off  block_type=register
  Register4 : xbsIndex_r4/Register  init=0  rst=off  en=on  dbl_ovrd=off  block_type=register
  Register5 : xbsIndex_r4/Register  init=0  rst=off  en=on  dbl_ovrd=off  block_type=register
  Register6 : xbsIndex_r4/Register  init=0  rst=off  en=off  dbl_ovrd=off  block_type=register
  Reinterpret2 : xbsIndex_r4/Reinterpret  force_arith_type=off  arith_type=Unsigned  force_bin_pt=off  bin_pt=18  block_type=reinterpret
  Reinterpret3 : xbsIndex_r4/Reinterpret  force_arith_type=off  arith_type=Unsigned  force_bin_pt=off  bin_pt=19  block_type=reinterpret
  ST9 : Subsystem
  TDDM_tbt_cordic : Subsystem
  Terminator : Terminator
  Terminator1 : Terminator
  Terminator2 : Terminator
  Up Sample : xbsIndex_r4/Up Sample  sample_ratio=R_tbt  copy_samples=off  en=off  latency=0  dbl_ovrd=off  block_type=usamp
  Up Sample1 : xbsIndex_r4/Up Sample  sample_ratio=R_tbt  copy_samples=on  en=off  latency=0  dbl_ovrd=off  block_type=usamp
  Up Sample2 : xbsIndex_r4/Up Sample  sample_ratio=R_tbt  copy_samples=on  en=off  latency=0  dbl_ovrd=off  block_type=usamp
  Up Sample3 : xbsIndex_r4/Up Sample  sample_ratio=R_tbt  copy_samples=on  en=off  latency=0  dbl_ovrd=off  block_type=usamp
  WaveScope : xbsIndex_r4/WaveScope  block_type=wavescope
  rect2pol : xbsIndex_r4/CORDIC 5.0   functional_selection=Translate  architectural_configuration=Word_Serial  pipelining_mode=Optimal  data_format=SignedFraction  phase_format=Radians  input_width=25  output_width=24  round_mode=Nearest_Even  iterations=0  precision=0  compensation_scaling=Embedded_Multiplier  coarse_rotation=on  aclken=off  aresetn=off  out_tready=off  cartesian_has_tuser=on  cartesian_has_tlast=off  cartesian_tuser_width=1  phase_has_tuser=off  phase_has_tlast=off  phase_tuser_width=1  out_tlast_behv=Null  flow_control=NonBlocking  optimize_goal=Resources  trim_axipin_name=on  ip_name=CORDIC  ip_version=5.0  dsptool_ready=true  ipcore_usecache=true  ipcore_useipmodelcache=true  wrapper_available=true  port_translation_map={ 'aclken' => 'en', 'aresetn' => 'rst' }  block_type=cordic_v5_0
      settings: infoedit=CORDIC 5.0
  tbt_amp_ch0_o : xbsIndex_r4/Gateway Out  inherit_from_input=on  hdl_port=on  timing_constraint=Data Rate  locs_specified=off  LOCs={}  UseAsDAC=off  DACChannel='1'  block_type=gatewayout
      settings: infoedit="Gateway out block.  Converts Xilinx fixed-point or floating-point type inputs into ouputs of type Simulink integer, single, double, or fixed point.<br><br>Hardware notes:  In hardware these blocks become top level output ports or are discarded, depending on how they are configured."
  tbt_amp_ch1_o : xbsIndex_r4/Gateway Out  inherit_from_input=off  hdl_port=on  timing_constraint=Data Rate  locs_specified=off  LOCs={}  UseAsDAC=off  DACChannel='1'  block_type=gatewayout
      settings: infoedit="Gateway out block.  Converts Xilinx fixed-point or floating-point type inputs into ouputs of type Simulink integer, single, double, or fixed point.<br><br>Hardware notes:  In hardware these blocks become top level output ports or are discarded, depending on how they are configured."
  tbt_amp_scope : Scope  NumInputPorts=2
      settings: TimeRange=0.00011214  YMin=0.38~0.184  YMax=0.55~0.208  SaveName=ScopeData19  MaxDataPoints=1000000  SampleInput=on
  tbt_pha_ch0_o : xbsIndex_r4/Gateway Out  inherit_from_input=on  hdl_port=on  timing_constraint=Data Rate  locs_specified=off  LOCs={}  UseAsDAC=off  DACChannel='1'  block_type=gatewayout
      settings: infoedit="Gateway out block.  Converts Xilinx fixed-point or floating-point type inputs into ouputs of type Simulink integer, single, double, or fixed point.<br><br>Hardware notes:  In hardware these blocks become top level output ports or are discarded, depending on how they are configured."
  tbt_pha_ch1_o : xbsIndex_r4/Gateway Out  inherit_from_input=off  hdl_port=on  timing_constraint=Data Rate  locs_specified=off  LOCs={}  UseAsDAC=off  DACChannel='1'  block_type=gatewayout
      settings: infoedit="Gateway out block.  Converts Xilinx fixed-point or floating-point type inputs into ouputs of type Simulink integer, single, double, or fixed point.<br><br>Hardware notes:  In hardware these blocks become top level output ports or are discarded, depending on how they are configured."
  amp_out : Outport
  phase_out : Outport  Port=2
  valid_out : Outport  Port=3
  ch_out : Outport  Port=4
  wires:
  Register4/1 -> Down Sample1/1
  Register5/1 -> Down Sample2/1
  Register6/1 -> Down Sample3/1
  Reinterpret2/1 -> Register4/1
  Reinterpret3/1 -> Register5/1
  valid_in/1 -> Up Sample/1
  Q_in/1 -> Up Sample1/1
  I_in/1 -> ST9/1(In), Up Sample2/1
  [tbt_cordic_amp_out] -> TDDM_tbt_cordic/1(tbt_cordic_din)
  [tbt_cordic_ch_out] -> TDDM_tbt_cordic/3(tbt_cordic_ch_in)
  ch_in/1 -> Up Sample3/1
  Register1/1 -> Down Sample4/1
  tbt_amp_ch0_o/1 -> tbt_amp_scope/1
  tbt_amp_ch1_o/1 -> tbt_amp_scope/2
  TDDM_tbt_cordic/1(tbt_cordic_data0_out) -> tbt_amp_ch0_o/1
  TDDM_tbt_cordic/2(tbt_cordic_data1_out) -> tbt_amp_ch1_o/1
  [tbt_cordic_phase_out] -> TDDM_tbt_cordic/2(tbt_cordic_pin)
  TDDM_tbt_cordic/3(tbt_cordic_phase0_out) -> tbt_pha_ch0_o/1
  TDDM_tbt_cordic/4(tbt_cordic_phase1_out) -> tbt_pha_ch1_o/1
  tbt_pha_ch0_o/1 -> Terminator/1
  tbt_pha_ch1_o/1 -> Terminator1/1
  rect2pol/2 -> Register6/1, Register4/2, Register5/2, Register1/2  "valid_out"
  rect2pol/3 -> Reinterpret2/1  "phase"
  rect2pol/4 -> Reinterpret3/1  "real"
  rect2pol/5 -> Register1/1  "ch_out"
  rect2pol/1 -> Terminator2/1  "ready"
  Up Sample/1 -> rect2pol/1  "valid_in"
  Up Sample1/1 -> rect2pol/2  "Q"
  Up Sample2/1 -> rect2pol/3  "I"
  Up Sample3/1 -> rect2pol/4  "ch_in"
  Down Sample3/1 -> Assert8/1
  Assert8/1 -> valid_out/1, [tbt_cordic_valid_out]  "p_valid_out"
  Down Sample1/1 -> Assert1/1
  Down Sample2/1 -> Assert2/1
  Down Sample4/1 -> Assert3/1
  Assert1/1 -> phase_out/1, [tbt_cordic_phase_out]  "p_phase_out"
  Assert2/1 -> amp_out/1, [tbt_cordic_amp_out]  "p_amp_out"
  Assert3/1 -> ch_out/1, [tbt_cordic_ch_out]  "p_ch_out"
